simulink model "Openloop_DC_motor_offline"  (R2022a)
settings: Solver=FixedStepDiscrete  StartTime=0.0  StopTime=0.02  FixedStep=0.000001  RelTol=1e-3
InitFcn:
  | Ts = 1e-4;
libraries: spsIGBTDiodeLib x12, spsSeriesRLCBranchLib x9, spsDCVoltageSourceLib x9, spsDCMachineLib x3, simulink x3, spspowerguiLib x3
settings Model: Creator=XCY  LastModifiedBy=Administrator
settings SolverCC: AlgebraicLoopSolver=TrustRegion
settings DataIOCC: ReturnWorkspaceOutputs=off
settings DebuggingCC: UnconnectedInputMsg=warning  UnconnectedOutputMsg=warning  UnconnectedLineMsg=warning  SFMachineParentedDataDiag=warning  ArithmeticOperatorsInVariantConditions=warning
settings SFSimCC: SimCustomHeaderCode="#include \"fuzzy.h\""  SimUserSources=fuzzy.c  SimUseLocalCustomCode=off  CustomCodeUndefinedFunction=UseInterfaceOnly
settings RTWCC: RTWUseLocalCustomCode=off
settings CodeAppCC: StateflowObjectComments=on
settings SimscapeCC: SimscapeNormalizeSystem=off

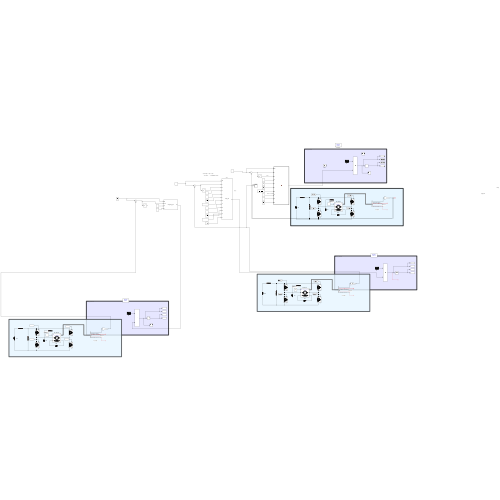
[thumbnail: Simulink's stored preview of the top-level diagram]
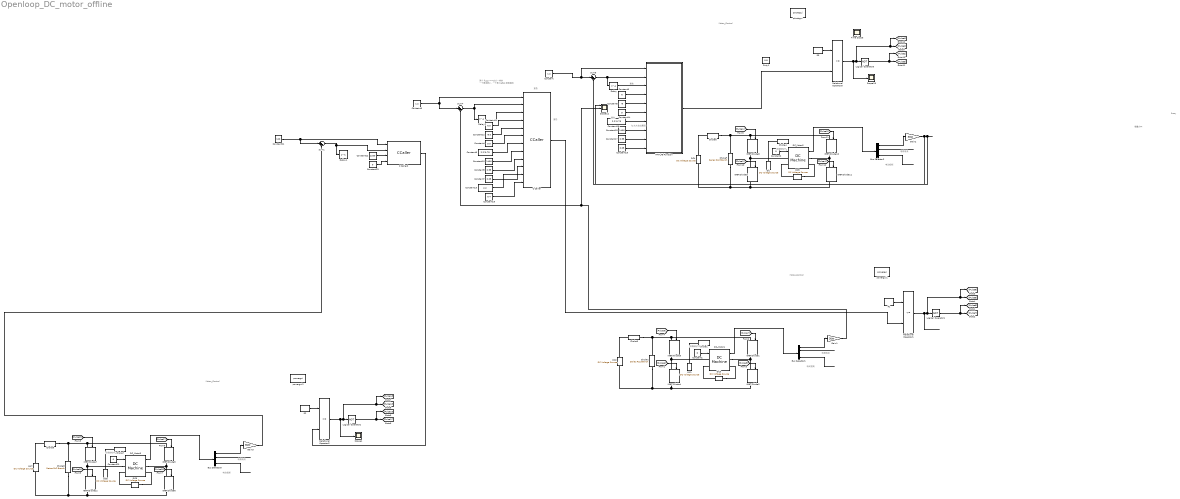
== system Openloop_DC_motor_offline ==
  note: 负载转矩TL
  note: 负载转矩TL
  note: k2太大会出震荡
  note: 两个 fuzzy——pid 一样的
      | 一个是调用c，一个是matlab语言编写
  note: 黄色
  note: 蓝色
  note: 电枢电流
  note: 电动扭矩
  note: fuzzy
  note: 增量式PI
  note: Motor_Control
  note: Motor_Control
  note: 电动扭矩
  note: 电枢电流
  note: 蓝色
  note: 黄色
  note: 电动扭矩
  note: 负载转矩TL
  note: Motor_Control
  note: 电枢电流
  Bus Selector1 : BusSelector  OutputSignals=Speed wm (rad/s),Armature current ia (A),Field current if (A),Electrical torque Te (n m)
  Bus Selector2 : BusSelector  OutputSignals=Speed wm (rad/s),Armature current ia (A),Field current if (A),Electrical torque Te (n m)
  Bus Selector3 : BusSelector  OutputSignals=Speed wm (rad/s),Armature current ia (A),Field current if (A),Electrical torque Te (n m)
  C Caller : CCaller  FunctionName=fuzzy_pid  PortSpecificationStruct="%)30     .    F!4   8    (     @         %    \"     T    !     0         %  0 \"0    $    _    07)G3F%M90  4&]R=$YA;64 4V-O<&4     26YD97@     5'EP90      4VEZ90      27-';&]B86P   X    P    !@    @    $          4    (     0    ,    !         !   P!O=70 #@   #     &    \"     0         !0    @    !     P    $         $  # &]U=  .    .     8    (    !          %    \"     $    &     0         0   ...(+7082 chars)"
  C Caller2 : CCaller  FunctionName=zengliang_pid  PortSpecificationStruct="%)30     .    J @   8    (     @         %    \"     4    !     0         %  0 \"0    $    _    07)G3F%M90  4&]R=$YA;64 4V-O<&4     26YD97@     5'EP90      4VEZ90      27-';&]B86P   X    P    !@    @    $          4    (     0    ,    !         !   P!O=70 #@   #     &    \"     0         !0    @    !     P    $         $  # &]U=  .    .     8    (    !          %    \"     $    &     0         0   ...(+2605 chars)"
  Choke{1,3..4,6..7,9} (6 alike) : spsSeriesRLCBranchLib/Series RLC Branch  LConnTagsString=__new0  RConnTagsString=__new0  BranchType=R  Resistance=5e-3  Inductance=2e-3  SetiL0=off  InitialCurrent=0  Capacitance=1e-6  Setx0=off  InitialVoltage=0  Measurements=None
  Choke2 : spsSeriesRLCBranchLib/Series RLC Branch  LConnTagsString=__new0  RConnTagsString=__new0  BranchType=C  Resistance=5e-3  Inductance=2e-3  SetiL0=off  InitialCurrent=0  Capacitance=1e-6  Setx0=off  InitialVoltage=0  Measurements=None
  Choke5 : spsSeriesRLCBranchLib/Series RLC Branch  LConnTagsString=__new0  RConnTagsString=__new0  BranchType=C  Resistance=5e-3  Inductance=2e-3  SetiL0=off  InitialCurrent=0  Capacitance=1e-6  Setx0=off  InitialVoltage=0  Measurements=None
  Choke8 : spsSeriesRLCBranchLib/Series RLC Branch  LConnTagsString=__new0  RConnTagsString=__new0  BranchType=C  Resistance=5e-3  Inductance=2e-3  SetiL0=off  InitialCurrent=0  Capacitance=1e-6  Setx0=off  InitialVoltage=0  Measurements=None
  Constant : Constant  Value=1.2
  Constant1 : Constant  Value=0
  Constant10 : Constant  Value=1400  OutDataTypeStr=Inherit: Inherit via back propagation
  Constant11 : Constant  Value=6.0  OutDataTypeStr=Inherit: Inherit via back propagation
  Constant12 : Constant  Value=-5.0
  Constant13 : Constant  Value=2.2  OutDataTypeStr=Inherit: Inherit via back propagation
  Constant14 : Constant  Value=5  OutDataTypeStr=Inherit: Inherit via back propagation
  Constant15 : Constant  Value=0.05  OutDataTypeStr=Inherit: Inherit via back propagation
  Constant16 : Constant  Value=2.2*0.75  OutDataTypeStr=Inherit: Inherit via back propagation
  Constant17 : Constant  Value=0.95  OutDataTypeStr=Inherit: Inherit via back propagation
  Constant18 : Constant  Value=1400  OutDataTypeStr=Inherit: Inherit via back propagation
  Constant19 : Constant  Value=0.4  OutDataTypeStr=Inherit: Inherit via back propagation
  Constant2 : Constant  Value=0
  Constant20 : Constant  Value=0
  Constant21 : Constant  Value=120
  Constant22 : Constant  Value=1200  OutDataTypeStr=Inherit: Inherit via back propagation
  Constant23 : Constant  Value=0  OutDataTypeStr=Inherit: Inherit via back propagation
  Constant3 : Constant  Value=1.2
  Constant4 : Constant  Value=5.0  OutDataTypeStr=Inherit: Inherit via back propagation
  Constant5 : Constant  Value=6  OutDataTypeStr=Inherit: Inherit via back propagation
  Constant6 : Constant  Value=-5
  Constant7 : Constant  Value=0.05  OutDataTypeStr=Inherit: Inherit via back propagation
  Constant8 : Constant  Value=2.2*0.75  OutDataTypeStr=Inherit: Inherit via back propagation
  Constant9 : Constant  Value=0.95  OutDataTypeStr=Inherit: Inherit via back propagation
  DC{,1..2,4,6..7} (6 alike) : spsDCVoltageSourceLib/DC Voltage Source  Amplitude=600  Measurements=None
  DC3 : spsDCVoltageSourceLib/DC Voltage Source  Amplitude=240  Measurements=None
  DC5 : spsDCVoltageSourceLib/DC Voltage Source  Amplitude=240  Measurements=None
  DC8 : spsDCVoltageSourceLib/DC Voltage Source  Amplitude=240  Measurements=None
  DC_Motor1 : spsDCMachineLib/DC Machine  PresetModel=No  MechanicalLoad=Torque TL  FieldType=Wound  ShowDetailedParameters=on  MeasurementBus=off  RLa="[ 0.6  0.012]"  RLf="[ 240  120]"  Laf=1.8  MachineConstant=Torque constant (N.m/A)  Ke=1.8  Kt=1.8  J=1  Bm=0.1  Tf=0  w0=0  Ifinit=1  TsPowergui=0  TsBlock=-1
      settings: AttributesFormatString=\n
  DC_Motor2 : spsDCMachineLib/DC Machine  PresetModel=No  MechanicalLoad=Torque TL  FieldType=Wound  ShowDetailedParameters=on  MeasurementBus=off  RLa="[ 0.6  0.012]"  RLf="[ 240  120]"  Laf=1.8  MachineConstant=Torque constant (N.m/A)  Ke=1.8  Kt=1.8  J=1  Bm=0.1  Tf=0  w0=0  Ifinit=1  TsPowergui=0  TsBlock=-1
      settings: AttributesFormatString=\n
  DC_Motor3 : spsDCMachineLib/DC Machine  PresetModel=No  MechanicalLoad=Torque TL  FieldType=Wound  ShowDetailedParameters=on  MeasurementBus=off  RLa="[ 0.6  0.012]"  RLf="[ 240  120]"  Laf=1.8  MachineConstant=Torque constant (N.m/A)  Ke=1.8  Kt=1.8  J=1  Bm=0.1  Tf=0  w0=0  Ifinit=1  TsPowergui=0  TsBlock=-1
      settings: AttributesFormatString=\n
  Delay : Delay  DelayLength=1
  Delay1 : Delay  DelayLength=1
  Delay2 : Delay  DelayLength=1
  Duty1 : Constant  Value=0.8
  Gain1 : Gain  Gain=30/pi
  Gain2 : Gain  Gain=30/pi
  Gain3 : Gain  Gain=30/pi
  IGBT/Diode{1..12} (12 alike) : spsIGBTDiodeLib/IGBT//Diode  Ron=1e-3  Rs=1e5  Cs=inf  Measurements=on
  Logical Operator1 : Logic  Operator=NOT  AllPortsSameDT=off  OutDataTypeStr=boolean
  Logical Operator2 : Logic  Operator=NOT  AllPortsSameDT=off  OutDataTypeStr=boolean
  Logical Operator3 : Logic  Operator=NOT  AllPortsSameDT=off  OutDataTypeStr=boolean
  MATLAB Function : MATLAB Function  TreatAsAtomicUnit=on
      settings: MinAlgLoopOccurrences=on
  R1 : simulink/Sources/Repeating Sequence  rep_seq_t=[0 0.00005 0.0001]  rep_seq_y=[0 1 0]
  R2 : simulink/Sources/Repeating Sequence  rep_seq_t=[0 0.00005 0.0001]  rep_seq_y=[0 1 0]
  R3 : simulink/Sources/Repeating Sequence  rep_seq_t=[0 0.00005 0.0001]  rep_seq_y=[0 1 0]
  Relational Operator1 : RelationalOperator  Operator=<=  OutDataTypeStr=boolean  RndMeth=Simplest  InputSameDT=off
  Relational Operator2 : RelationalOperator  Operator=<=  OutDataTypeStr=boolean  RndMeth=Simplest  InputSameDT=off
  Relational Operator3 : RelationalOperator  Operator=<=  OutDataTypeStr=boolean  RndMeth=Simplest  InputSameDT=off
  Scope1 : Scope
  Scope12 : Scope  NumInputPorts=3
  Scope15 : Scope
  Sum1 : Sum  Inputs=|+-
  Sum4 : Sum  Inputs=|+-
  Sum5 : Sum  Inputs=|+-
  Time Scope : Scope
  powergui : spspowerguiLib/powergui  Priority=1  SimulationMode=Discrete  SampleTime=0.000001  frequency=60  Iterations=50  frequencyindice=0  Pbase=100e6  ErrMax=1e-4  UnitsV=kV  UnitsW=MW  buscounter=0  FunctionMessages=off  echomessages=off  EnableUseOfTLC=off  CurrentSourceSwitches=off  DisableSnubberDevices=off  DisableRonSwitches=off  DisableVfSwitches=off  DisplayEquations=off  AutomaticDiscreteSolvers=off  SolverType=Tustin/Backward Euler (TBE)  Interpol=off  ExternalGateDelay=off  methode=off  Ts=100  x0status=blocks  SPID=off  SwTol=0  HookPort=off  NonlinearTolerance=1e-4  nMaxIteration=100  ContinueOnMaxIteration=off  RestoreLinks=warning  ResistiveCurrentMeasurement=off  Frange=[0:2:500]  Ylog=off  Xlog=on  ShowGrid=off  save=off  variable=ZData  structure=0  ZoomFFT=off  StartTime=0.0  cycles=1  DisplayStyle=1  fundamental=60  FreqAxis=off  MaxFrequency=1000  frequencyindicesteady=1  RmsSteady=1  display=off
  powergui1 : spspowerguiLib/powergui  Priority=1  SimulationMode=Discrete  SampleTime=1e-6  frequency=60  Iterations=50  frequencyindice=0  Pbase=100e6  ErrMax=1e-4  UnitsV=kV  UnitsW=MW  buscounter=0  FunctionMessages=off  echomessages=off  EnableUseOfTLC=off  CurrentSourceSwitches=off  DisableSnubberDevices=off  DisableRonSwitches=off  DisableVfSwitches=off  DisplayEquations=off  AutomaticDiscreteSolvers=off  SolverType=Tustin/Backward Euler (TBE)  Interpol=off  ExternalGateDelay=off  methode=off  Ts=100  x0status=blocks  SPID=off  SwTol=0  HookPort=off  NonlinearTolerance=1e-4  nMaxIteration=100  ContinueOnMaxIteration=off  RestoreLinks=warning  ResistiveCurrentMeasurement=off  Frange=[0:2:500]  Ylog=off  Xlog=on  ShowGrid=off  save=off  variable=ZData  structure=0  ZoomFFT=off  StartTime=0.0  cycles=1  DisplayStyle=1  fundamental=60  FreqAxis=off  MaxFrequency=1000  frequencyindicesteady=1  RmsSteady=1  display=off
  powergui2 : spspowerguiLib/powergui  Priority=1  SimulationMode=Discrete  SampleTime=1e-6  frequency=60  Iterations=50  frequencyindice=0  Pbase=100e6  ErrMax=1e-4  UnitsV=kV  UnitsW=MW  buscounter=0  FunctionMessages=off  echomessages=off  EnableUseOfTLC=off  CurrentSourceSwitches=off  DisableSnubberDevices=off  DisableRonSwitches=off  DisableVfSwitches=off  DisplayEquations=off  AutomaticDiscreteSolvers=off  SolverType=Tustin/Backward Euler (TBE)  Interpol=off  ExternalGateDelay=off  methode=off  Ts=100  x0status=blocks  SPID=off  SwTol=0  HookPort=off  NonlinearTolerance=1e-4  nMaxIteration=100  ContinueOnMaxIteration=off  RestoreLinks=warning  ResistiveCurrentMeasurement=off  Frange=[0:2:500]  Ylog=off  Xlog=on  ShowGrid=off  save=off  variable=ZData  structure=0  ZoomFFT=off  StartTime=0.0  cycles=1  DisplayStyle=1  fundamental=60  FreqAxis=off  MaxFrequency=1000  frequencyindicesteady=1  RmsSteady=1  display=off
  wires:
  Delay/1 -> MATLAB Function/3(e1)
  Constant18/1 -> MATLAB Function/8(ku)
  Constant17/1 -> MATLAB Function/9(as)
  Constant5/1 -> MATLAB Function/4(N)
  Constant16/1 -> MATLAB Function/7(k2)
  Constant14/1 -> MATLAB Function/6(b)
  Constant6/1 -> MATLAB Function/5(a)
  Constant15/1 -> MATLAB Function/10(ao)
  Sum5/1 -> Delay/1, MATLAB Function/2(e)
  [Pulse4] -> IGBT/Diode11/1
  [Pulse2] -> IGBT/Diode9/1
  Relational Operator3/1 -> Logical Operator3/1, [Pulse1], [Pulse4], Scope15/1
  Logical Operator3/1 -> [Pulse3], [Pulse2]
  [Pulse1] -> IGBT/Diode8/1
  DC_Motor2/1 -> Bus Selector2/1
  Constant2/1 -> DC_Motor2/1
  [Pulse3] -> IGBT/Diode10/1
  Bus Selector2/1 -> Gain2/1  "<Speed wm (rad/s)>"
  Bus Selector2/2 -> ?  "<Armature current ia (A)>"
  Bus Selector2/4 -> ?  "<Electrical torque Te (n m)>"
  MATLAB Function/1(y) -> Relational Operator3/2
  Relational Operator1/1 -> Logical Operator1/1, [Pulse5], [Pulse8]
  Logical Operator1/1 -> [Pulse7], [Pulse6]
  DC_Motor1/1 -> Bus Selector1/1
  [Pulse5] -> IGBT/Diode3/1
  [Pulse7] -> IGBT/Diode1/1
  Bus Selector1/1 -> Gain1/1  "<Speed wm (rad/s)>"
  Bus Selector1/4 -> ?  "<Electrical torque Te (n m)>"
  Bus Selector1/2 -> ?  "<Armature current ia (A)>"
  [Pulse6] -> IGBT/Diode4/1
  Constant1/1 -> DC_Motor1/1
  [Pulse8] -> IGBT/Diode2/1
  Sum4/1 -> C Caller/2, Delay2/1
  Gain1/1 -> Scope12/2, Sum4/2
  Delay2/1 -> C Caller/3
  Constant9/1 -> C Caller/9
  Constant8/1 -> C Caller/7
  Constant10/1 -> C Caller/8
  Constant3/1 -> Sum4/1, C Caller/1
  Constant7/1 -> C Caller/10
  Constant4/1 -> C Caller/6
  Constant12/1 -> C Caller/5
  Constant11/1 -> C Caller/4
  C Caller/1 -> Relational Operator1/2
  R3/1 -> Relational Operator3/1
  R1/1 -> Relational Operator1/1
  Constant/1 -> MATLAB Function/1(Ma), Sum5/1
  Gain2/1 -> Sum5/2, Scope12/1
  Constant13/1 -> C Caller/11
  Constant19/1 -> C Caller/12
  Bus Selector3/4 -> ?  "<Electrical torque Te (n m)>"
  Constant20/1 -> DC_Motor3/1
  [Pulse17] -> IGBT/Diode5/1
  [Pulse16] -> IGBT/Diode12/1
  DC_Motor3/1 -> Bus Selector3/1
  Bus Selector3/2 -> ?  "<Armature current ia (A)>"
  Bus Selector3/1 -> Gain3/1  "<Speed wm (rad/s)>"
  Relational Operator2/1 -> Scope1/1, Logical Operator2/1, [Pulse15], [Pulse18]
  [Pulse18] -> IGBT/Diode6/1
  [Pulse15] -> IGBT/Diode7/1
  Logical Operator2/1 -> [Pulse17], [Pulse16]
  Constant21/1 -> C Caller2/1, Sum1/1
  Sum1/1 -> C Caller2/2, Delay1/1
  Gain3/1 -> Sum1/2
  Constant22/1 -> C Caller2/3
  Constant23/1 -> C Caller2/4
  R2/1 -> Relational Operator2/1
  C Caller2/1 -> Relational Operator2/2
  connections:
  DC/RConn1 -- Choke4/LConn1
  IGBT/Diode10/LConn1 -- IGBT/Diode8/LConn1 -- Choke6/RConn1 -- Choke5/LConn1
  IGBT/Diode10/RConn1 -- IGBT/Diode11/LConn1 -- DC_Motor2/RConn1
  DC4/LConn1 -- IGBT/Diode9/RConn1 -- IGBT/Diode11/RConn1 -- Choke5/RConn1
  IGBT/Diode9/LConn1 -- IGBT/Diode8/RConn1 -- DC_Motor2/LConn1
  DC5/RConn1 -- DC_Motor2/LConn2
  DC5/LConn1 -- DC_Motor2/RConn2
  DC4/RConn1 -- Choke6/LConn1
  IGBT/Diode4/LConn1 -- IGBT/Diode3/RConn1 -- DC_Motor1/LConn1
  DC2/LConn1 -- Choke2/RConn1 -- IGBT/Diode4/RConn1 -- IGBT/Diode2/RConn1
  Choke2/LConn1 -- Choke3/RConn1 -- IGBT/Diode3/LConn1 -- IGBT/Diode1/LConn1
  IGBT/Diode1/RConn1 -- IGBT/Diode2/LConn1 -- DC_Motor1/RConn1
  DC2/RConn1 -- Choke3/LConn1
  DC3/RConn1 -- DC_Motor1/LConn2
  DC3/LConn1 -- DC_Motor1/RConn2
  DC1/RConn1 -- Choke1/LConn1
  IGBT/Diode6/RConn1 -- DC7/LConn1 -- Choke8/RConn1 -- IGBT/Diode12/RConn1
  DC_Motor3/RConn1 -- IGBT/Diode5/RConn1 -- IGBT/Diode6/LConn1
  IGBT/Diode5/LConn1 -- Choke8/LConn1 -- Choke9/RConn1 -- IGBT/Diode7/LConn1
  DC_Motor3/LConn1 -- IGBT/Diode12/LConn1 -- IGBT/Diode7/RConn1
  DC8/RConn1 -- DC_Motor3/LConn2
  DC6/RConn1 -- Choke7/LConn1
  DC8/LConn1 -- DC_Motor3/RConn2
  DC7/RConn1 -- Choke9/LConn1

== matlab function Openloop_DC_motor_offline/MATLAB Function ==
  data: Ma input; e input; e1 input; N input; y output; a input; b input; k2 input; ku input; as input; ao input
function y= fuzyy_pid(Ma,e,e1,N,a,b,k2,ku,as,ao)


	ed = e - e1;
	E = -(2 * N) * (e * k2 - (a + b)) / (b - a);    
	E1 = E;
	EC = -(2 * N) * (ed - (a + b)) / (b - a);
	EC1 = 270 * EC;
	a1 = (1.0 / N) * (as - ao) * abs(E1) + ao;
	y= (-(a1 * E1 + (1 - a1) * EC1) / 2)*ku*Ma;
end
    %y=ku;
